simulink model "simexa29"  (Simulink 4.00)
settings: Solver=ode45  SolverMode=SingleTasking  StartTime=0.0  StopTime=5.0  RelTol=1e-5  AbsTol=1e-6
settings Model: LastModifiedBy=saadat  LimitDataPoints=off  RTWTemplateMakefile=grt_vc.tmf  ExtModeTrigMode=oneshot  ExtModeArmWhenConnect=off

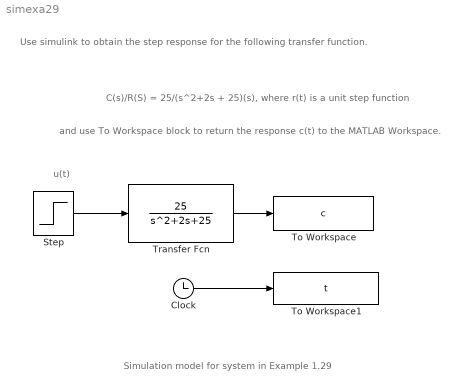
== system simexa29 ==
  note: Simulation model for system in Example 1.29
  note: C(s)/R(S) = 25/(s^2+2s + 25)(s), where r(t) is a unit step function
  note: Use simulink to obtain the step response for the
      |    following transfer function.
  note: and use To Workspace block to return the response c(t) to the
      | MATLAB Workspace.
  note: u(t)
  Clock : Clock
      settings: DisplayTime=off  Decimation=10
  Step : Step  Time=0  Before=0  After=1  SampleTime=0
  To Workspace : ToWorkspace  VariableName=c  SampleTime=-1  SaveFormat=Array
  To Workspace1 : ToWorkspace  VariableName=t  SampleTime=-1  SaveFormat=Array
  Transfer Fcn : TransferFcn  Numerator=[25]  Denominator="[1  2   25]"  AbsoluteTolerance=auto  Realization=auto
  wires:
  Clock/1 -> To Workspace1/1
  Step/1 -> Transfer Fcn/1
  Transfer Fcn/1 -> To Workspace/1
